simulink model "Top_Level_System"  (R2018b)
settings: Solver=FixedStepAuto  StartTime=0.0  StopTime=10.0  RelTol=1e-3
values from neighbouring files (symbols this model uses):
  SRC_Ts = 0.001    [Parameters.m]
settings Model: Creator=univ4123  LastModifiedBy=univ4123
settings RTWCC: GenCodeOnly=on  Toolchain=MinGW64 | gmake (64-bit Windows)  BuildConfiguration=Faster Runs

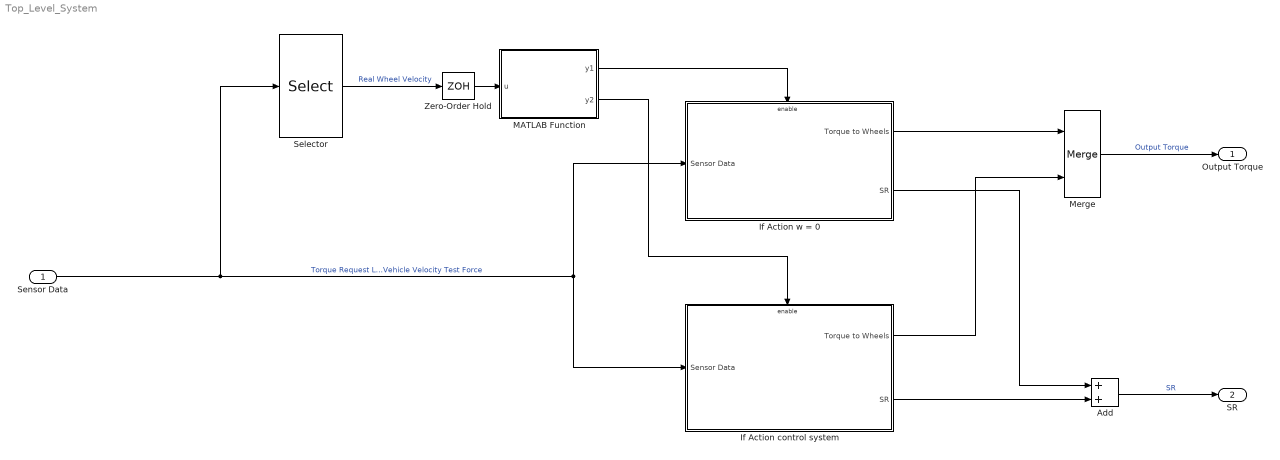
== system Top_Level_System ==
  Sensor Data : Inport
  Add : Sum
  If Action control system : Subsystem  TreatAsAtomicUnit=on
  If Action w = 0 : Subsystem  TreatAsAtomicUnit=on
  MATLAB Function : MATLAB Function  TreatAsAtomicUnit=on
  Merge : Merge
  Selector : Selector  InputPortWidth=5  IndexOptions=Index vector (dialog)  Indices=[2 3]  OutputSizes=1
  Zero-Order Hold : ZeroOrderHold  SampleTime=SRC_Ts
  Output Torque : Outport
  SR : Outport  Port=2
  wires:
  Zero-Order Hold/1 -> MATLAB Function/1(u)
  Selector/1 -> Zero-Order Hold/1  "Real Wheel Velocity"
  MATLAB Function/2(y2) -> If Action control system/Enable
  MATLAB Function/1(y1) -> If Action w = 0/Enable
  If Action control system/2(SR) -> Add/2
  If Action w = 0/2(SR) -> Add/1
  If Action control system/1(Torque to Wheels) -> Merge/2
  Sensor Data/1 -> Selector/1, If Action control system/1(Sensor Data), If Action w = 0/1(Sensor Data)  "Torque Request Left Wheel Velocity Right Wheel Velocity True Vehicle Velocity Test Force"
  Merge/1 -> Output Torque/1  "Output Torque"
  Add/1 -> SR/1  "SR"
  If Action w = 0/1(Torque to Wheels) -> Merge/1

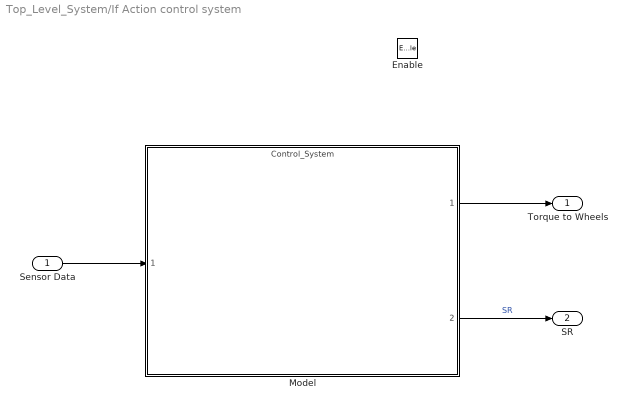
== system Top_Level_System/If Action control system ==
  Sensor Data : Inport
  Enable : EnablePort
  Model : ModelReference  ModelNameDialog=Control_System.slx  SimulationMode=Normal  ModelReferenceVersion=1.33
  Torque to Wheels : Outport
  SR : Outport  Port=2
  wires:
  Sensor Data/1 -> Model/1
  Model/1 -> Torque to Wheels/1
  Model/2 -> SR/1  "SR"

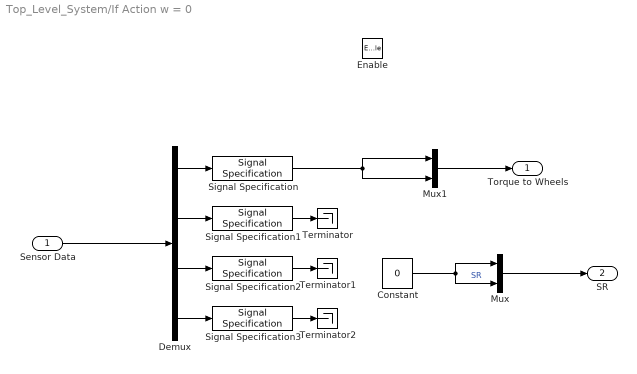
== system Top_Level_System/If Action w = 0 ==
  Sensor Data : Inport
  Enable : EnablePort
  Constant : Constant  Value=0  SampleTime=SRC_Ts
  Demux : Demux
  Mux : Mux  Inputs=2
  Mux1 : Mux  Inputs=2
  Signal Specification : SignalSpecification  Dimensions=1
  Signal Specification1 : SignalSpecification  Dimensions=2
  Signal Specification2 : SignalSpecification  Dimensions=1
  Signal Specification3 : SignalSpecification  Dimensions=1
  Terminator : Terminator
  Terminator1 : Terminator
  Terminator2 : Terminator
  Torque to Wheels : Outport
  SR : Outport  Port=2
  wires:
  Constant/1 -> Mux/2, Mux/1  "SR"
  Sensor Data/1 -> Demux/1
  Demux/1 -> Signal Specification/1
  Demux/2 -> Signal Specification1/1
  Demux/3 -> Signal Specification2/1
  Mux/1 -> SR/1
  Signal Specification2/1 -> Terminator1/1
  Signal Specification1/1 -> Terminator/1
  Signal Specification/1 -> Mux1/2, Mux1/1
  Mux1/1 -> Torque to Wheels/1
  Signal Specification3/1 -> Terminator2/1
  Demux/4 -> Signal Specification3/1

== matlab function Top_Level_System/MATLAB Function ==
  data: u input; y1 output; y2 output
function [y1,y2] = Active(u)
y1=0;
y2=0;

if any(u) == 0
    y1 = 1;
else
    y2 = 1;
end
